simulink model "d2_model_2015"  (R2021a)
settings: Solver=VariableStepAuto  StartTime=0.0  StopTime=40  RelTol=1e-3
values from neighbouring files (symbols this model uses):
  A = [0 1 0 0; -K_m/M 0 K_m/M 0; 0 0 0 1; K_m/M 0 -K_m/M 0]    [d2.m]
  Ao = [Ai zeros(3, 3); zeros(3, 3) Ai]    [d2.m]
  At = [A B*Co; zeros(6, 4) Ao]    [d2.m]
  B = [0 0; 1/M 0; 0 0; 0 1/M]    [d2.m]
  Bo = [Bi zeros(3, 1); zeros(3, 1) Bi]    [d2.m]
  Bt = [B zeros(4, 2); zeros(6, 2) Bo]    [d2.m]
  C = [1 0 0 0; 0 0 1 0]    [d2.m]
  Co = [Ci zeros(1, 3); zeros(1, 3) Ci]    [d2.m]
  Ct = [C zeros(2, 6)]    [d2.m]
  Do = zeros(2, 2)    [d2.m]
  Ft = -K    [d2.m]
  Kt = H'    [d2.m]
  r = [1;1]    [d2.m]
settings Model: Creator=Murillo  LastModifiedBy=Murillo

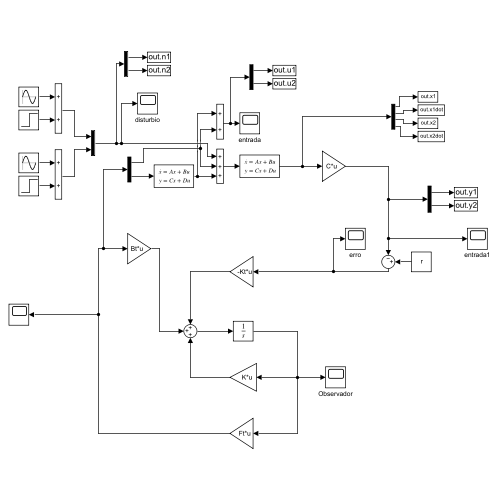
[thumbnail: Simulink's stored preview of the top-level diagram]
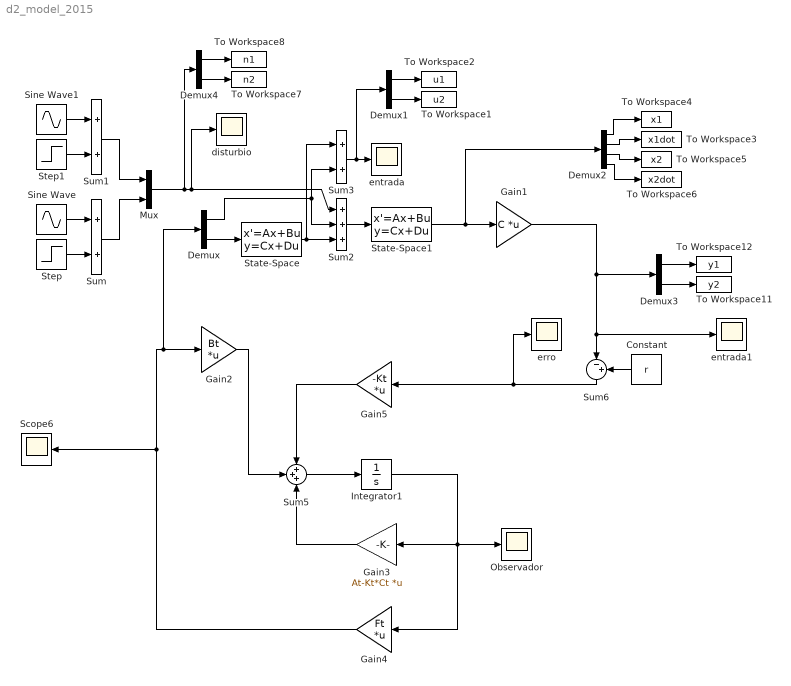
== system d2_model_2015 ==
  Constant : Constant  Value=r
  Demux{,1,3..4} (4 alike) : Demux  Outputs=2
  Demux2 : Demux
  Gain1 : Gain  Gain=C  Multiplication=Matrix(K*u)
  Gain2 : Gain  Gain=Bt  Multiplication=Matrix(K*u)
  Gain3 : Gain  Gain=At-Kt*Ct  Multiplication=Matrix(K*u)
  Gain4 : Gain  Gain=Ft  Multiplication=Matrix(K*u)
  Gain5 : Gain  Gain=-Kt  Multiplication=Matrix(K*u)
  Integrator1 : Integrator
  Mux : Mux  Inputs=2
  Observador : Scope
  Scope6 : Scope
  Sine Wave : Sin  Frequency=2  Phase=pi/2  SampleTime=0
  Sine Wave1 : Sin  Amplitude=2  Frequency=2  Phase=pi  SampleTime=0
  State-Space : StateSpace  A=Ao  B=Bo  C=Co  D=Do  InitialCondition=0
  State-Space1 : StateSpace  A=A  B=B  C=eye(4)  D=[0 0; 0 0; 0 0; 0 0]  InitialCondition=0
  Step : Step  SampleTime=0
  Step1 : Step  SampleTime=0
  Sum : Sum
  Sum1 : Sum
  Sum2 : Sum  Inputs=+++
  Sum3 : Sum
  Sum5 : Sum  Inputs=+++
  Sum6 : Sum  Inputs=|-+
  To Workspace1 : ToWorkspace  VariableName=u2  SampleTime=-1
      settings: Save2DSignal=2-D array (concatenate along first dimension)
  To Workspace11 : ToWorkspace  VariableName=y2  SampleTime=-1
      settings: Save2DSignal=2-D array (concatenate along first dimension)
  To Workspace12 : ToWorkspace  VariableName=y1  SampleTime=-1
      settings: Save2DSignal=2-D array (concatenate along first dimension)
  To Workspace2 : ToWorkspace  VariableName=u1  SampleTime=-1
      settings: Save2DSignal=2-D array (concatenate along first dimension)
  To Workspace3 : ToWorkspace  VariableName=x1dot  SampleTime=-1
      settings: Save2DSignal=2-D array (concatenate along first dimension)
  To Workspace4 : ToWorkspace  VariableName=x1  SampleTime=-1
      settings: Save2DSignal=2-D array (concatenate along first dimension)
  To Workspace5 : ToWorkspace  VariableName=x2  SampleTime=-1
      settings: Save2DSignal=2-D array (concatenate along first dimension)
  To Workspace6 : ToWorkspace  VariableName=x2dot  SampleTime=-1
      settings: Save2DSignal=2-D array (concatenate along first dimension)
  To Workspace7 : ToWorkspace  VariableName=n2  SampleTime=-1
      settings: Save2DSignal=2-D array (concatenate along first dimension)
  To Workspace8 : ToWorkspace  VariableName=n1  SampleTime=-1
      settings: Save2DSignal=2-D array (concatenate along first dimension)
  disturbio : Scope
  entrada : Scope
  entrada1 : Scope
  erro : Scope
  wires:
  Step/1 -> Sum/2
  Sine Wave/1 -> Sum/1
  Sine Wave1/1 -> Sum1/1
  Step1/1 -> Sum1/2
  Sum1/1 -> Mux/1
  Sum/1 -> Mux/2
  State-Space/1 -> Sum3/1, Sum2/3
  Demux/2 -> State-Space/1
  Demux/1 -> Sum2/2, Sum3/2
  Mux/1 -> Demux4/1, Sum2/1, disturbio/1
  Sum2/1 -> State-Space1/1
  Gain3/1 -> Sum5/3
  Integrator1/1 -> Gain3/1, Gain4/1, Observador/1
  Constant/1 -> Sum6/2
  Gain5/1 -> Sum5/1
  Gain2/1 -> Sum5/2
  Sum6/1 -> erro/1, Gain5/1
  Sum5/1 -> Integrator1/1
  Demux3/2 -> To Workspace11/1
  Demux3/1 -> To Workspace12/1
  Gain1/1 -> Demux3/1, entrada1/1, Sum6/1
  Demux2/4 -> To Workspace6/1
  Demux2/1 -> To Workspace4/1
  Demux2/2 -> To Workspace3/1
  Demux2/3 -> To Workspace5/1
  State-Space1/1 -> Demux2/1, Gain1/1
  Gain4/1 -> Gain2/1, Demux/1, Scope6/1
  Demux1/1 -> To Workspace2/1
  Demux1/2 -> To Workspace1/1
  Sum3/1 -> Demux1/1, entrada/1
  Demux4/2 -> To Workspace7/1
  Demux4/1 -> To Workspace8/1
